simulink model "lab_4_task_1_simulink"  (R2025b)
settings: Solver=ode4  StartTime=0.0  StopTime=10  FixedStep=0.1  RelTol=1e-3
values from neighbouring files (symbols this model uses):
  A0 = eye(3)    [lab_4_task_3.m]    (also in lab_5_task_1.m; lab_5_task_2.m = A312(phi0, theta0, psi0))
  I = diag([ix iy iz])    [lab_3_task_3.m]    (also in lab_4_task_3.m; lab_5_task_1.m; lab_5_task_2.m; lab_6_task_1.m = diag([ ix iy iz ]))
  w0 = [0.01 0.01 0.01]    [lab_3_task_3.m]    (also in lab_4_task_3.m = [wx0 wy0 wz0]; lab_5_task_1.m = [wx0 wy0 wz0]; lab_5_task_2.m = [wx0; wy0; wz0;]; lab_6_task_1.m = [wx0 wy0 wz0])
libraries: matrix_library x1
settings Model: Creator=nicol  LastModifiedBy=nicol

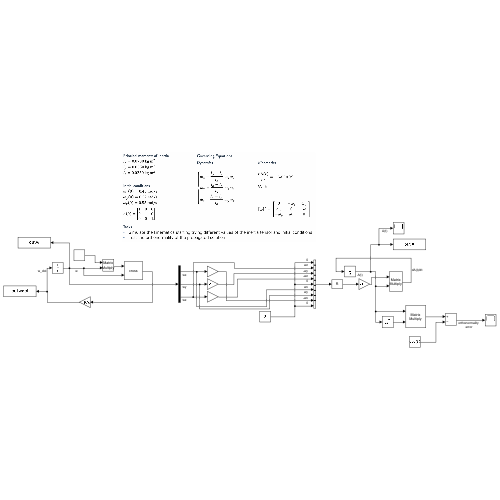
[thumbnail: Simulink's stored preview of the top-level diagram]
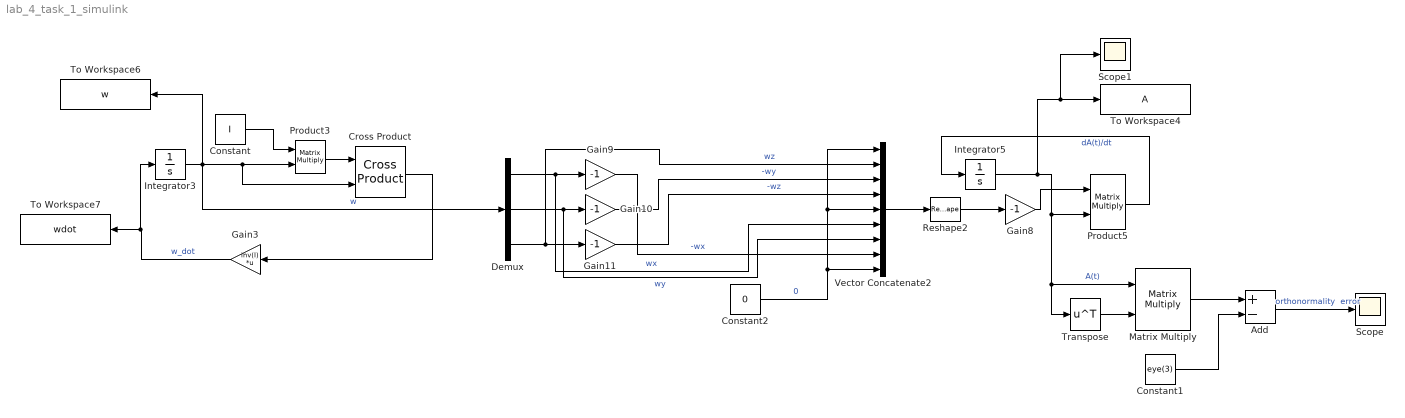
== system lab_4_task_1_simulink ==
  Add : Sum  Inputs=+-
  Constant : Constant  Value=I
  Constant1 : Constant  Value=eye(3)
  Constant2 : Constant  Value=0
  Cross Product : matrix_library/Cross Product
  Demux : Demux  Outputs=3
  Gain{8..11} (4 alike) : Gain  Gain=-1
  Gain3 : Gain  Gain=inv(I)  Multiplication=Matrix(K*u)
  Integrator3 : Integrator  InitialCondition=w0
  Integrator5 : Integrator  InitialCondition=A0
  Matrix Multiply : Product  Multiplication=Matrix(*)
  Product3 : Product  Multiplication=Matrix(*)
  Product5 : Product  Multiplication=Matrix(*)
  Reshape2 : Reshape  OutputDimensionality=Customize  OutputDimensions=[3,3]
  Scope : Scope
      settings: ActiveDisplayYMinimum=-0.00024619045043009456  ActiveDisplayYMaximum=0.00014018276145496243
  Scope1 : Scope
      settings: ActiveDisplayYMinimum=-1.248054944065039  ActiveDisplayYMaximum=1.2497838826738932
  To Workspace4 : ToWorkspace  VariableName=A  SaveFormat=Timeseries  SampleTime=-1
  To Workspace6 : ToWorkspace  VariableName=w  SaveFormat=Timeseries  SampleTime=-1
  To Workspace7 : ToWorkspace  VariableName=wdot  SaveFormat=Timeseries  SampleTime=-1
  Transpose : Math  Operator=transpose
  Vector Concatenate2 : Concatenate  NumInputs=9
  wires:
  Product3/1 -> Cross Product/1
  Integrator3/1 -> Demux/1, Cross Product/2, Product3/2, To Workspace6/1  "w"
  Constant/1 -> Product3/1
  Cross Product/1 -> Gain3/1
  Gain3/1 -> Integrator3/1, To Workspace7/1  "w_dot"
  Reshape2/1 -> Gain8/1
  Gain8/1 -> Product5/1
  Integrator5/1 -> Scope1/1, To Workspace4/1, Product5/2, Transpose/1, Matrix Multiply/1  "A(t)"
  Product5/1 -> Integrator5/1  "dA(t)/dt"
  Vector Concatenate2/1 -> Reshape2/1
  Demux/1 -> Vector Concatenate2/6, Gain9/1  "wx"
  Demux/2 -> Vector Concatenate2/7, Gain10/1  "wy"
  Demux/3 -> Vector Concatenate2/2, Gain11/1  "wz"
  Constant2/1 -> Vector Concatenate2/1, Vector Concatenate2/5, Vector Concatenate2/9  "0"
  Gain10/1 -> Vector Concatenate2/3  "-wy"
  Gain11/1 -> Vector Concatenate2/4  "-wz"
  Gain9/1 -> Vector Concatenate2/8  "-wx"
  Transpose/1 -> Matrix Multiply/2
  Matrix Multiply/1 -> Add/1
  Constant1/1 -> Add/2
  Add/1 -> Scope/1  "orthonormality  error"
